simulink model "Analysis_model"  (R2025b)
settings: Solver=VariableStepAuto  StartTime=0.0  StopTime=10.0  RelTol=1e-3
values from neighbouring files (symbols this model uses):
  DZ = 0.35    [Stabilization.m]
  KI = (time_const/Km)*w_cl^2    [Stabilization.m]
  Km = 1300    [Stabilization.m]    (also in Stabilization_Mod.m = 1)
  KP = (2*w_cl*zeta_cl*time_const - 1)/Km    [Stabilization.m]
undefined symbols (not defined in the file or in its folder): DiscIntNeverNeededParam, SATURATION, time_const, Ts
settings Model: Creator=ohyus  LastModifiedBy=ohyus

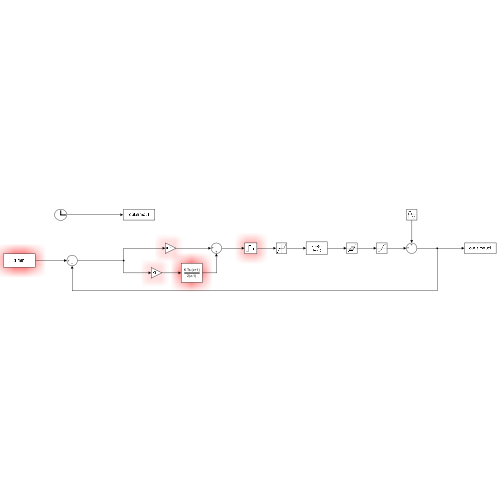
[thumbnail: Simulink's stored preview of the top-level diagram]
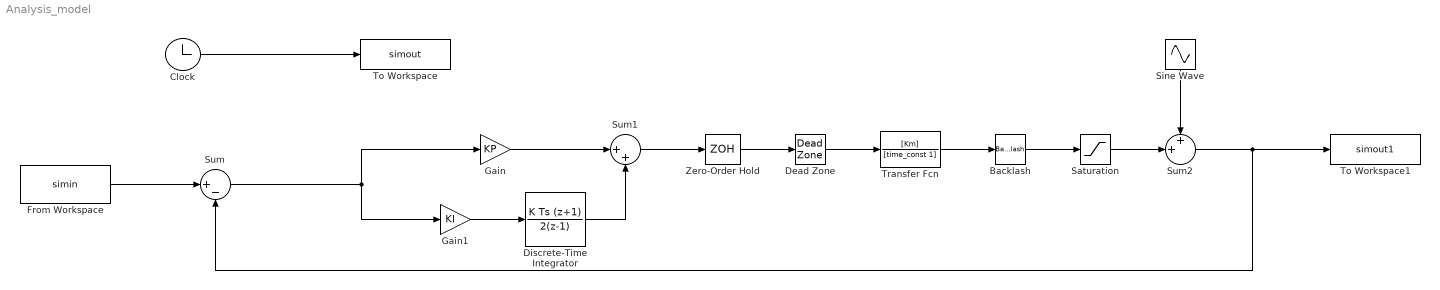
== system Analysis_model ==
  Backlash : Backlash
  Clock : Clock
  Dead Zone : DeadZone  LowerValue=DZ  UpperValue=-DZ
  Discrete-Time Integrator : DiscreteIntegrator  IntegratorMethod=Integration: Trapezoidal  SampleTime=Ts  ICPrevOutput=DiscIntNeverNeededParam  ICPrevScaledInput=DiscIntNeverNeededParam
  From Workspace : FromWorkspace  VariableName=simin
  Gain : Gain  Gain=KP
  Gain1 : Gain  Gain=KI
  Saturation : Saturate  UpperLimit=SATURATION  LowerLimit=-SATURATION
  Sine Wave : Sin  Frequency=0.5*2*pi  SampleTime=0
  Sum : Sum  Inputs=|+-
  Sum1 : Sum  Inputs=|++
  Sum2 : Sum  Inputs=++|
  To Workspace : ToWorkspace  VariableName=simout  SaveFormat=Timeseries  SampleTime=-1
  To Workspace1 : ToWorkspace  VariableName=simout1  SaveFormat=Timeseries  SampleTime=-1
  Transfer Fcn : TransferFcn  Numerator=[Km]  Denominator=[time_const 1]
  Zero-Order Hold : ZeroOrderHold  SampleTime=Ts
  wires:
  Clock/1 -> To Workspace/1
  Sum/1 -> Gain1/1, Gain/1
  Gain/1 -> Sum1/1
  Gain1/1 -> Discrete-Time Integrator/1
  From Workspace/1 -> Sum/1
  Sum1/1 -> Zero-Order Hold/1
  Dead Zone/1 -> Transfer Fcn/1
  Transfer Fcn/1 -> Backlash/1
  Backlash/1 -> Saturation/1
  Saturation/1 -> Sum2/2
  Discrete-Time Integrator/1 -> Sum1/2
  Zero-Order Hold/1 -> Dead Zone/1
  Sine Wave/1 -> Sum2/1
  Sum2/1 -> Sum/2, To Workspace1/1
